simulink model "test_model_2018a2"  (R2018a)
settings: Solver=VariableStepAuto  StartTime=0.0  StopTime=4  RelTol=1e-3
values from neighbouring files (symbols this model uses):
  A = sys_d.A    [discreteTest.m]    (also in discreteTestAttacked.m)
  B = sys_d.B    [discreteTest.m]    (also in discreteTestAttacked.m)
  C = sys_d.C    [discreteTest.m]    (also in discreteTestAttacked.m)
  K = [   5.261, -0.023 ... (first row only)    [discreteTest.m]    (also in discreteTestAttacked.m)
  steeringAngle = zeros(1, time)    [discreteTest.m]    (also in discreteTestAttacked.m)
  Ts = 0.04    [discreteTest.m]    (also in discreteTestAttacked.m)
undefined symbols (not defined in the file or in its folder): canChannel, L
libraries: canlib x6, simulink x6, canmsglib x4, hdlsllib x4
settings Model: Creator=Shreyash  LastModifiedBy=Shreyash

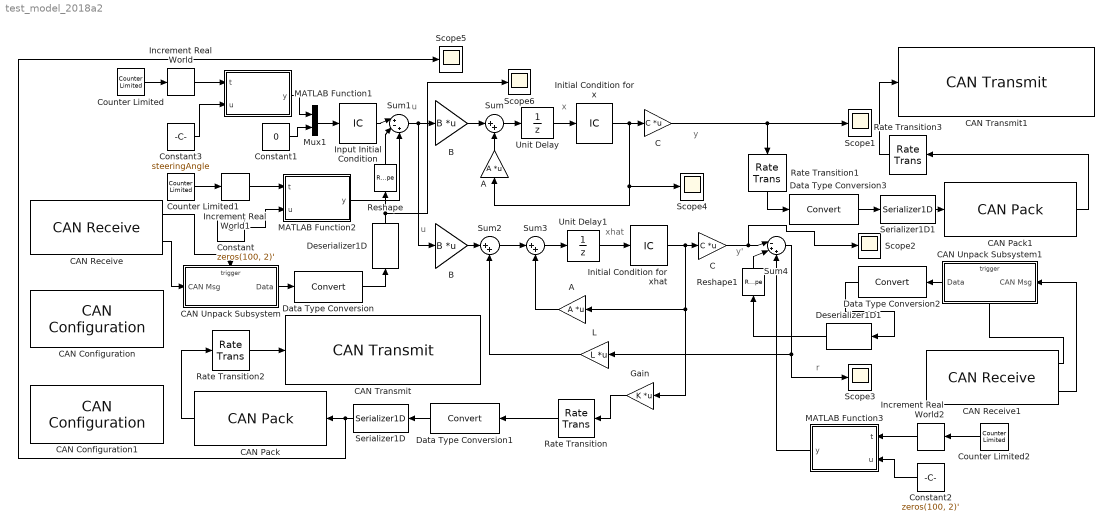
== system test_model_2018a2 ==
  note: y
  note: r
  note: y'
  note: u
  note: u
  note: x
  note: xhat
  A : Gain  Gain=A  Multiplication=Matrix(K*u)
  "A " : Gain  Gain=A  Multiplication=Matrix(K*u)
  B : Gain  Gain=B  Multiplication=Matrix(K*u)
  "B " : Gain  Gain=B  Multiplication=Matrix(K*u)
  C : Gain  Gain=C  Multiplication=Matrix(K*u)
  "C " : Gain  Gain=C  Multiplication=Matrix(K*u)
  CAN Configuration : canlib/CAN Configuration  BlockHandle=11.0001  DeviceMenu=MathWorks Virtual 1 (Channel 1)  Device=MathWorks Virtual 1 (Channel 1)  ObjConstructor=canChannel('MathWorks','Virtual 1',1)  BusSpeed=500000  EnableBitParameters=off  AckMode=Normal
      settings: SourceProductName=Vehicle Network Toolbox  SourceProductBaseCode=VN
  CAN Configuration1 : canlib/CAN Configuration  BlockHandle=12.0001  DeviceMenu=MathWorks Virtual 1 (Channel 2)  Device=MathWorks Virtual 1 (Channel 2)  ObjConstructor=canChannel('MathWorks','Virtual 1',2)  BusSpeed=500000  EnableBitParameters=off  AckMode=Normal
      settings: SourceProductName=Vehicle Network Toolbox  SourceProductBaseCode=VN
  CAN Pack : canmsglib/CAN Pack  MsgList=(none)  MsgName=CAN Msg  MsgIDType=Standard (11-bit identifier)  MsgIdentifier=100  MsgLength=8  SignalInfo=signal$0$64$1$4$1$0$1$0$-Inf$Inf$#  NSignals=1  StartBits=str2num('[int32(0)]')  SignalSizes=str2num('[int32(64)]')  ByteOrders=str2num('[int32(1)]')  DataTypes=str2num('[int32(4)]')  MultiplexTypes=str2num('[int32(1)]')  MultiplexValues=str2num('[double(0)]')  Factors=str2num('[double(1)]')  Offsets=str2num('[double(0)]')  Minimums=str2num('[double(-Inf)]')  Maximums=str2num('[double(Inf)]')  Remote=off  ApplyMinMax=off  BusOutput=off
      settings: SourceProductName=Vehicle Network Toolbox  SourceProductBaseCode=VN  DataFormat=manually specified signals
  CAN Pack1 : canmsglib/CAN Pack  MsgList=(none)  MsgName=CAN Msg  MsgIDType=Standard (11-bit identifier)  MsgIdentifier=100  MsgLength=8  SignalInfo=signal$0$64$1$4$1$0$1$0$-Inf$Inf$#  NSignals=1  StartBits=str2num('[int32(0)]')  SignalSizes=str2num('[int32(64)]')  ByteOrders=str2num('[int32(1)]')  DataTypes=str2num('[int32(4)]')  MultiplexTypes=str2num('[int32(1)]')  MultiplexValues=str2num('[double(0)]')  Factors=str2num('[double(1)]')  Offsets=str2num('[double(0)]')  Minimums=str2num('[double(-Inf)]')  Maximums=str2num('[double(Inf)]')  Remote=off  ApplyMinMax=off  BusOutput=off
      settings: SourceProductName=Vehicle Network Toolbox  SourceProductBaseCode=VN  DataFormat=manually specified signals
  CAN Receive : canlib/CAN Receive  BlockHandle=15.0001  DeviceMenu=MathWorks Virtual 1 (Channel 2)  Device=MathWorks Virtual 1 (Channel 2)  ObjConstructor=canChannel('MathWorks','Virtual 1',2)  EnableStandardIDsFilter=off  StandardIDs=100  EnableExtendedIDsFilter=off  ExtendedIDs=0  SampleTime=0.01  MsgsPerTimestep=all  StdIDsCombo=Allow only  ExtIDsCombo=Block all  InternalFilterUpdateStatus=on  BusOutput=off
      settings: SourceProductName=Vehicle Network Toolbox  SourceProductBaseCode=VN
  CAN Receive1 : canlib/CAN Receive  BlockHandle=16.0001  DeviceMenu=MathWorks Virtual 1 (Channel 2)  Device=MathWorks Virtual 1 (Channel 2)  ObjConstructor=canChannel('MathWorks','Virtual 1',2)  EnableStandardIDsFilter=off  StandardIDs=100  EnableExtendedIDsFilter=off  ExtendedIDs=0  SampleTime=0.01  MsgsPerTimestep=all  StdIDsCombo=Allow only  ExtIDsCombo=Block all  InternalFilterUpdateStatus=on  BusOutput=off
      settings: SourceProductName=Vehicle Network Toolbox  SourceProductBaseCode=VN
  CAN Transmit : canlib/CAN Transmit  BlockHandle=17.0001  DeviceMenu=MathWorks Virtual 1 (Channel 1)  Device=MathWorks Virtual 1 (Channel 1)  ObjConstructor=canChannel('MathWorks','Virtual 1',1)  EnablePeriodicTransmit=off  MessagePeriod=0.04
      settings: SourceProductName=Vehicle Network Toolbox  SourceProductBaseCode=VN
  CAN Transmit1 : canlib/CAN Transmit  BlockHandle=18.0001  DeviceMenu=MathWorks Virtual 1 (Channel 1)  Device=MathWorks Virtual 1 (Channel 1)  ObjConstructor=canChannel('MathWorks','Virtual 1',1)  EnablePeriodicTransmit=off  MessagePeriod=0.04
      settings: SourceProductName=Vehicle Network Toolbox  SourceProductBaseCode=VN
  CAN Unpack Subsystem : Subsystem  TreatAsAtomicUnit=on
  CAN Unpack Subsystem1 : Subsystem  TreatAsAtomicUnit=on
  Constant : Constant  Value=zeros(100, 2)'
  Constant1 : Constant  Value=0
  Constant2 : Constant  Value=zeros(100, 2)'
  Constant3 : Constant  Value=steeringAngle  SampleTime=0.04
  Counter Limited : simulink/Sources/Counter Limited  uplimit=124  tsamp=0.04
  Counter Limited1 : simulink/Sources/Counter Limited  uplimit=99  tsamp=0.04
  Counter Limited2 : simulink/Sources/Counter Limited  uplimit=99  tsamp=0.04
  Data Type Conversion : DataTypeConversion  SaturateOnIntegerOverflow=on
  Data Type Conversion1 : DataTypeConversion
  Data Type Conversion2 : DataTypeConversion  SaturateOnIntegerOverflow=on
  Data Type Conversion3 : DataTypeConversion
  Deserializer1D : hdlsllib/HDL Operations/Deserializer1D  Ratio=2  IdleCycles=10000  InitialCondition=0  startIn=off  validIn=off  validOut=off  inputDataDimensions=[1]  inputSampleTime=-1  inputSignalType=auto
      settings: SourceProductName=HDL Coder  SourceProductBaseCode=HD
  Deserializer1D1 : hdlsllib/HDL Operations/Deserializer1D  Ratio=2  IdleCycles=98  InitialCondition=0  startIn=off  validIn=off  validOut=off  inputDataDimensions=[1]  inputSampleTime=-1  inputSignalType=auto
      settings: SourceProductName=HDL Coder  SourceProductBaseCode=HD
  Gain : Gain  Gain=K  Multiplication=Matrix(K*u)
  Increment Real World : simulink/Additional Math & Discrete/Additional Math: Increment - Decrement/Increment Real World
      settings: SourceProductName=Simulink  SourceProductBaseCode=SL
  Increment Real World1 : simulink/Additional Math & Discrete/Additional Math: Increment - Decrement/Increment Real World
      settings: SourceProductName=Simulink  SourceProductBaseCode=SL
  Increment Real World2 : simulink/Additional Math & Discrete/Additional Math: Increment - Decrement/Increment Real World
      settings: SourceProductName=Simulink  SourceProductBaseCode=SL
  Initial Condition for x : InitialCondition  Value=[0;0]
  Initial Condition for xhat : InitialCondition  Value=[0;0]
  Input Initial Condition : InitialCondition  Value=[0;0]
  L : Gain  Gain=L  Multiplication=Matrix(K*u)
  MATLAB Function1 : MATLAB Function  TreatAsAtomicUnit=on
  MATLAB Function2 : MATLAB Function  TreatAsAtomicUnit=on
  MATLAB Function3 : MATLAB Function  TreatAsAtomicUnit=on
  Mux1 : Mux  Inputs=2
  Rate Transition : RateTransition  Integrity=off  Deterministic=off  InitialCondition=Ts  OutPortSampleTime=Ts
  Rate Transition1 : RateTransition  Integrity=off  Deterministic=off  InitialCondition=Ts  OutPortSampleTime=Ts
  Rate Transition2 : RateTransition  Deterministic=off  OutPortSampleTimeMultiple=0.01  OutPortSampleTime=.0001
  Rate Transition3 : RateTransition  Deterministic=off  OutPortSampleTime=0.01
  Reshape : Reshape  OutputDimensionality=Customize  OutputDimensions=[2,1]
  Reshape1 : Reshape  OutputDimensionality=Customize  OutputDimensions=[2,1]
  Scope{1..6} (6 alike) : Scope
  Serializer1D : hdlsllib/HDL Operations/Serializer1D  Ratio=2  IdleCycles=2  validIn=off  startOut=off  validOut=off  inputDataDimensions=[2,1]  inputSampleTime=-1  inputSignalType=auto
      settings: SourceProductName=HDL Coder  SourceProductBaseCode=HD
  Serializer1D1 : hdlsllib/HDL Operations/Serializer1D  Ratio=2  IdleCycles=2  validIn=off  startOut=off  validOut=off  inputDataDimensions=[2,1]  inputSampleTime=-1  inputSignalType=auto
      settings: SourceProductName=HDL Coder  SourceProductBaseCode=HD
  Sum : Sum  Inputs=|++
  Sum1 : Sum  Inputs=|+-+
  Sum2 : Sum  Inputs=|++
  Sum3 : Sum  Inputs=|++
  Sum4 : Sum  Inputs=|-++
  Unit Delay : UnitDelay  SampleTime=-1
  Unit Delay1 : UnitDelay  SampleTime=-1
  wires:
  "B "/1 -> Sum/1
  Unit Delay/1 -> Initial Condition for x/1
  Sum/1 -> Unit Delay/1
  "A "/1 -> Sum/2
  Constant1/1 -> Mux1/2
  B/1 -> Sum2/1
  Sum2/1 -> Sum3/1
  Sum3/1 -> Unit Delay1/1
  Unit Delay1/1 -> Initial Condition for xhat/1
  L/1 -> Sum2/2
  A/1 -> Sum3/2
  Sum4/1 -> Scope3/1, L/1
  Initial Condition for x/1 -> "A "/1, Scope4/1, "C "/1
  C/1 -> Scope2/1, Sum4/1
  Initial Condition for xhat/1 -> A/1, Gain/1, C/1
  Sum1/1 -> B/1, "B "/1
  Mux1/1 -> Input Initial Condition/1
  Input Initial Condition/1 -> Sum1/1
  Gain/1 -> Rate Transition/1
  CAN Receive/2 -> CAN Unpack Subsystem/1(CAN Msg)
  CAN Receive/1 -> CAN Unpack Subsystem/Trigger
  Rate Transition/1 -> Data Type Conversion1/1
  CAN Receive1/2 -> CAN Unpack Subsystem1/1(CAN Msg)
  CAN Receive1/1 -> CAN Unpack Subsystem1/Trigger
  Constant3/1 -> MATLAB Function1/2(u)
  Counter Limited/1 -> Increment Real World/1
  Increment Real World/1 -> MATLAB Function1/1(t)
  MATLAB Function1/1(y) -> Mux1/1
  Counter Limited1/1 -> Increment Real World1/1
  Increment Real World1/1 -> MATLAB Function2/1(t)
  Counter Limited2/1 -> Increment Real World2/1
  Increment Real World2/1 -> MATLAB Function3/1(t)
  Constant/1 -> MATLAB Function2/2(u)
  Constant2/1 -> MATLAB Function3/2(u)
  MATLAB Function3/1(y) -> Sum4/3
  Rate Transition1/1 -> Data Type Conversion3/1
  MATLAB Function2/1(y) -> Sum1/3
  CAN Pack1/1 -> Rate Transition3/1
  "C "/1 -> Scope1/1, Rate Transition1/1
  CAN Unpack Subsystem/1(Data) -> Data Type Conversion/1
  CAN Unpack Subsystem1/1(Data) -> Data Type Conversion2/1
  Rate Transition3/1 -> CAN Transmit1/1
  CAN Pack/1 -> Rate Transition2/1
  Reshape/1 -> Sum1/2
  Data Type Conversion/1 -> Deserializer1D/1
  Deserializer1D/1 -> Scope6/1, Reshape/1
  Rate Transition2/1 -> CAN Transmit/1
  Data Type Conversion1/1 -> Serializer1D/1
  Serializer1D/1 -> Scope5/1, CAN Pack/1
  Reshape1/1 -> Sum4/2
  Deserializer1D1/1 -> Reshape1/1
  Data Type Conversion2/1 -> Deserializer1D1/1
  Data Type Conversion3/1 -> Serializer1D1/1
  Serializer1D1/1 -> CAN Pack1/1

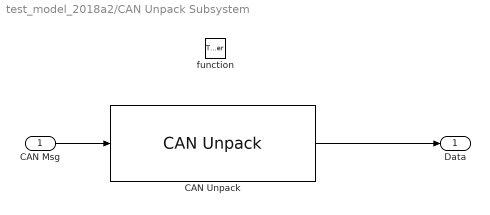
== system test_model_2018a2/CAN Unpack Subsystem ==
  CAN Msg : Inport
  function : TriggerPort  TriggerType=function-call  VariantControl=Variant
  CAN Unpack : canmsglib/CAN Unpack  MsgList=(none)  MsgName=CAN Msg  MsgIDType=Standard (11-bit identifier)  MsgIdentifier=100  MsgLength=8  SignalInfo=signal1$0$64$1$4$1$0$1$0$-Inf$Inf$#  NSignals=1  IDPort=off  TimestampPort=off  ErrorPort=off  RemotePort=off  LengthPort=off  StatusPort=off  StartBits=str2num('[int32(0)]')  SignalSizes=str2num('[int32(64)]')  ByteOrders=str2num('[int32(1)]')  DataTypes=str2num('[int32(4)]')  MultiplexTypes=str2num('[int32(1)]')  MultiplexValues=str2num('[double(0)]')  Factors=str2num('[double(1)]')  Offsets=str2num('[double(0)]')  Minimums=str2num('[double(-Inf)]')  Maximums=str2num('[double(Inf)]')  ApplyMinMax=off
      settings: SourceProductName=Vehicle Network Toolbox  SourceProductBaseCode=VN
  Data : Outport
  wires:
  CAN Msg/1 -> CAN Unpack/1
  CAN Unpack/1 -> Data/1

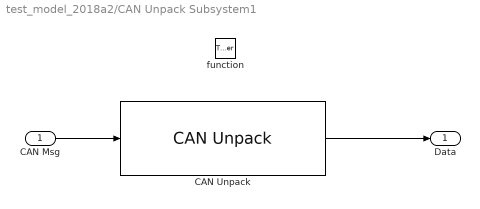
== system test_model_2018a2/CAN Unpack Subsystem1 ==
  CAN Msg : Inport
  function : TriggerPort  TriggerType=function-call  VariantControl=Variant
  CAN Unpack : canmsglib/CAN Unpack  MsgList=(none)  MsgName=CAN Msg  MsgIDType=Standard (11-bit identifier)  MsgIdentifier=100  MsgLength=8  SignalInfo=Signal1$0$64$1$4$1$0$1$0$-Inf$Inf$#  NSignals=1  IDPort=off  TimestampPort=off  ErrorPort=off  RemotePort=off  LengthPort=off  StatusPort=off  StartBits=str2num('[int32(0)]')  SignalSizes=str2num('[int32(64)]')  ByteOrders=str2num('[int32(1)]')  DataTypes=str2num('[int32(4)]')  MultiplexTypes=str2num('[int32(1)]')  MultiplexValues=str2num('[double(0)]')  Factors=str2num('[double(1)]')  Offsets=str2num('[double(0)]')  Minimums=str2num('[double(-Inf)]')  Maximums=str2num('[double(Inf)]')  ApplyMinMax=off
      settings: SourceProductName=Vehicle Network Toolbox  SourceProductBaseCode=VN
  Data : Outport
  wires:
  CAN Msg/1 -> CAN Unpack/1
  CAN Unpack/1 -> Data/1

== matlab function test_model_2018a2/MATLAB Function1 ==
  data: t input; u input; y output
function y = fcn(t, u)
y = u(t)*(pi/180)*0.0625;
%for t = 1 :100
    %y = au(:, t);
    %y = (-1 + 2.*rand(1, 2))'; 
end

== matlab function test_model_2018a2/MATLAB Function2 ==
  data: t input; u input; y output
function y = fcn(t, u)
y = u(:, t);
%for t = 1 :100
    %y = au(:, t);
    %y = (-1 + 2.*rand(1, 2))'; 
end

== matlab function test_model_2018a2/MATLAB Function3 ==
  data: t input; u input; y output
function y = fcn(t, u)
y = u(:, t);
%for t = 1 :100
    %y = au(:, t);
    %y = (-1 + 2.*rand(1, 2))'; 
end
